simulink model "HammingTXRX"  (R2021a)
settings: Solver=VariableStepAuto  StartTime=0.0  StopTime=10.0  RelTol=1e-3
settings Model: Creator=FraH  LastModifiedBy=FraH

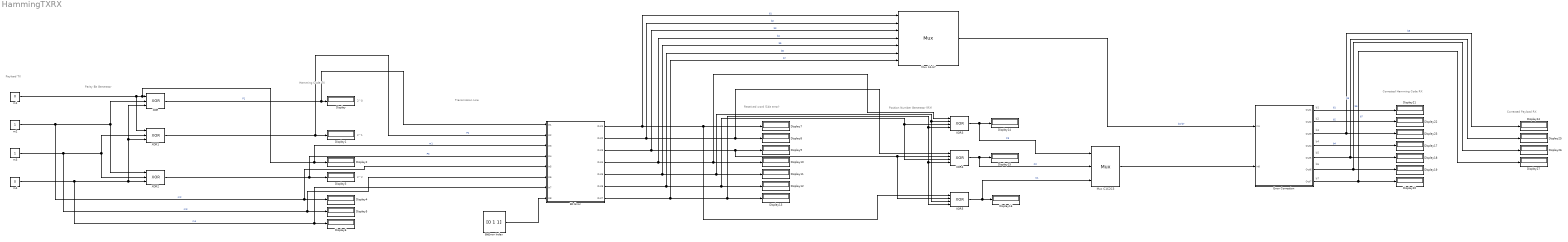
== system HammingTXRX ==
  note: b7
  note: b6
  note: b5
  note: b4
  note: b3
  note: b2
  note: b1
  note: 2^2
  note: 2^1
  note: 2^0
  note: Transmission Line
  note: Corrected Payload RX
  note: Corrected Hamming Code RX
  note: Received word (1bit error)
  note: Hamming Code TX
  note: Parity Bit Generator
  note: Payload TX
  note: Position Number Generator (RX)
  Bit Error : Subsystem
  BitError Index : Constant  Value=[0 1 1]  OutDataTypeStr=boolean
  Display{,1..27} (28 alike) : Display
  Error Correction : Subsystem
  Mux C1C2C3 : Mux  Inputs=3
  Mux b1-b7 : Mux  Inputs=7
  XOR : Logic  Operator=XOR  Inputs=3  AllPortsSameDT=off  OutDataTypeStr=boolean
  XOR1 : Logic  Operator=XOR  Inputs=3  AllPortsSameDT=off  OutDataTypeStr=boolean
  XOR2 : Logic  Operator=XOR  Inputs=3  AllPortsSameDT=off  OutDataTypeStr=boolean
  XOR3 : Logic  Operator=XOR  Inputs=4  AllPortsSameDT=off  OutDataTypeStr=boolean
  XOR4 : Logic  Operator=XOR  Inputs=4  AllPortsSameDT=off  OutDataTypeStr=boolean
  XOR5 : Logic  Operator=XOR  Inputs=4  AllPortsSameDT=off  OutDataTypeStr=boolean
  m1 : Constant  Value=0
  m2 : Constant
  m3 : Constant
  m4 : Constant  Value=0
  wires:
  m1/1 -> Bit Error/3(In3), Display2/1, XOR/1, XOR1/1  "m1"
  m2/1 -> Display4/1, Bit Error/5(In5), XOR2/1, XOR/2  "m2"
  m4/1 -> Bit Error/7(In7), Display6/1, XOR2/3, XOR1/3, XOR/3  "m4"
  m3/1 -> Display5/1, Bit Error/6(In6), XOR2/2, XOR1/2  "m3"
  XOR/1 -> Bit Error/1(In1), Display/1  "P1"
  XOR1/1 -> Bit Error/2(In2), Display1/1  "P2"
  XOR2/1 -> Display3/1, Bit Error/4(In4)  "P3"
  BitError Index/1 -> Bit Error/8(In8)
  Bit Error/1(Out1) -> Mux b1-b7/1, XOR5/1, Display7/1  "b1"
  Bit Error/2(Out2) -> Mux b1-b7/2, XOR4/1, Display8/1  "b2"
  Bit Error/3(Out3) -> Mux b1-b7/3, Display9/1, XOR4/2, XOR5/2  "b3"
  Bit Error/4(Out4) -> Mux b1-b7/4, XOR3/1, Display10/1  "b4"
  Bit Error/5(Out5) -> Mux b1-b7/5, XOR5/3, XOR3/2, Display11/1  "b5"
  Bit Error/6(Out6) -> Mux b1-b7/6, XOR4/3, XOR3/3, Display12/1  "b6"
  Bit Error/7(Out7) -> Mux b1-b7/7, XOR5/4, XOR4/4, XOR3/4, Display13/1  "b7"
  XOR3/1 -> Mux C1C2C3/1, Display14/1  "C3"
  XOR4/1 -> Mux C1C2C3/2, Display15/1  "C2"
  XOR5/1 -> Mux C1C2C3/3, Display16/1  "C1"
  Mux C1C2C3/1 -> Error Correction/2(In8)
  Mux b1-b7/1 -> Error Correction/1(In1)  "b1-b7"
  Error Correction/1(Out1) -> Display21/1  "b1"
  Error Correction/2(Out2) -> Display22/1  "b2"
  Error Correction/3(Out3) -> Display23/1, Display24/1  "b3"
  Error Correction/4(Out4) -> Display17/1  "b4"
  Error Correction/5(Out5) -> Display25/1, Display18/1  "b5"
  Error Correction/6(Out6) -> Display26/1, Display19/1  "b6"
  Error Correction/7(Out7) -> Display27/1, Display20/1  "b7"

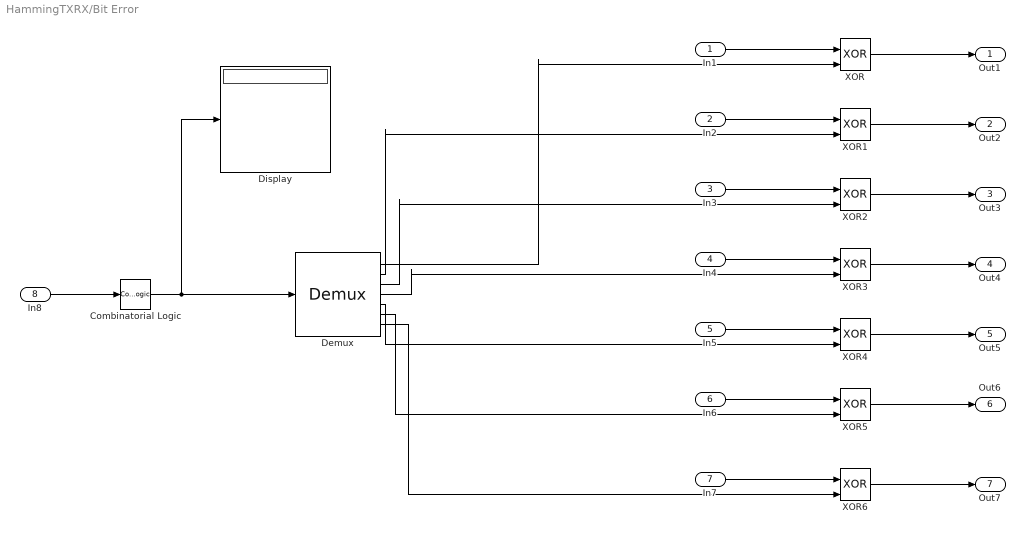
== system HammingTXRX/Bit Error ==
  In1 : Inport
  In2 : Inport  Port=2
  In3 : Inport  Port=3
  In4 : Inport  Port=4
  In5 : Inport  Port=5
  In6 : Inport  Port=6
  In7 : Inport  Port=7
  In8 : Inport  Port=8  OutDataTypeStr=boolean
  Combinatorial Logic : CombinatorialLogic  TruthTable=[0 0 0 0 0 0 0;1 0 0 0 0 0 0;0 1 0 0 0 0 0;0 0 1 0 0 0 0;0 0 0 1 0 0 0;0 0 0 0 1 0 0;0 0 0 0 0 1 0;0 0 0 0 0 0 1]
  Demux : Demux  Outputs=7
  Display : Display
  XOR{,1..6} (7 alike) : Logic  Operator=XOR  IconShape=distinctive  AllPortsSameDT=off  OutDataTypeStr=boolean
  Out1 : Outport
  Out2 : Outport  Port=2
  Out3 : Outport  Port=3
  Out4 : Outport  Port=4
  Out5 : Outport  Port=5
  Out6 : Outport  Port=6
  Out7 : Outport  Port=7
  wires:
  In1/1 -> XOR/1
  In2/1 -> XOR1/1
  In3/1 -> XOR2/1
  In4/1 -> XOR3/1
  In5/1 -> XOR4/1
  In6/1 -> XOR5/1
  In7/1 -> XOR6/1
  XOR/1 -> Out1/1
  XOR1/1 -> Out2/1
  XOR2/1 -> Out3/1
  XOR3/1 -> Out4/1
  XOR4/1 -> Out5/1
  XOR5/1 -> Out6/1
  XOR6/1 -> Out7/1
  In8/1 -> Combinatorial Logic/1
  Combinatorial Logic/1 -> Display/1, Demux/1
  Demux/1 -> XOR/2
  Demux/2 -> XOR1/2
  Demux/3 -> XOR2/2
  Demux/4 -> XOR3/2
  Demux/5 -> XOR4/2
  Demux/6 -> XOR5/2
  Demux/7 -> XOR6/2

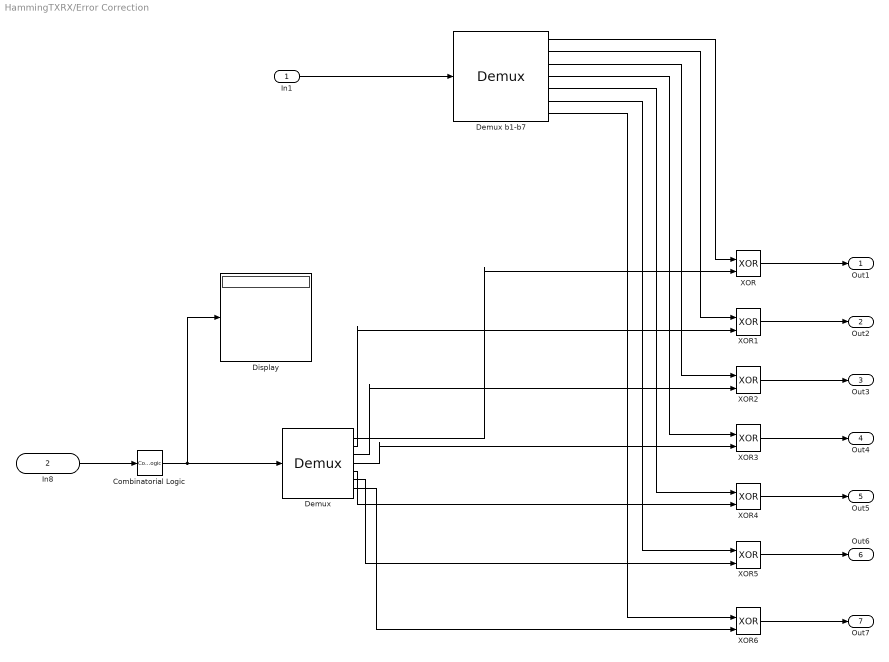
== system HammingTXRX/Error Correction ==
  In1 : Inport
  In8 : Inport  Port=2  OutDataTypeStr=boolean
  Combinatorial Logic : CombinatorialLogic  TruthTable=[0 0 0 0 0 0 0;1 0 0 0 0 0 0;0 1 0 0 0 0 0;0 0 1 0 0 0 0;0 0 0 1 0 0 0;0 0 0 0 1 0 0;0 0 0 0 0 1 0;0 0 0 0 0 0 1]
  Demux : Demux  Outputs=7
  Demux b1-b7 : Demux  Outputs=7
  Display : Display
  XOR{,1..6} (7 alike) : Logic  Operator=XOR  IconShape=distinctive  AllPortsSameDT=off  OutDataTypeStr=boolean
  Out1 : Outport
  Out2 : Outport  Port=2
  Out3 : Outport  Port=3
  Out4 : Outport  Port=4
  Out5 : Outport  Port=5
  Out6 : Outport  Port=6
  Out7 : Outport  Port=7
  wires:
  Demux b1-b7/2 -> XOR1/1
  Demux b1-b7/3 -> XOR2/1
  Demux b1-b7/4 -> XOR3/1
  XOR/1 -> Out1/1
  XOR1/1 -> Out2/1
  XOR2/1 -> Out3/1
  XOR3/1 -> Out4/1
  XOR4/1 -> Out5/1
  XOR5/1 -> Out6/1
  XOR6/1 -> Out7/1
  In8/1 -> Combinatorial Logic/1
  Combinatorial Logic/1 -> Display/1, Demux/1
  Demux/1 -> XOR/2
  Demux/2 -> XOR1/2
  Demux/3 -> XOR2/2
  Demux/4 -> XOR3/2
  Demux/5 -> XOR4/2
  Demux/6 -> XOR5/2
  Demux/7 -> XOR6/2
  In1/1 -> Demux b1-b7/1
  Demux b1-b7/1 -> XOR/1
  Demux b1-b7/5 -> XOR4/1
  Demux b1-b7/6 -> XOR5/1
  Demux b1-b7/7 -> XOR6/1
